simulink model "luenberger_obs2_w_design"  (R2023b)
settings: Solver=FixedStepAuto  StartTime=0.0  StopTime=T  FixedStep=dt  RelTol=1e-3
values from neighbouring files (symbols this model uses):
  A = [0 1 0 -1; -ks/mv -bs/mv 0 bs/mv; 0 0 0 1; ks/mr bs/mr -kp/mr -(bs+bp)/mr]    [define_system.m]
  A_sim_case = eval(sprintf('A_c    [design_cls.m]    (also in design_obs.m)
  B1 = [0; 0; -1; bp/mr]    [define_system.m]
  B1_sim_case = eval(sprintf('B1_c    [design_cls.m]    (also in design_obs.m)
  B2 = [0; 1/mv; 0; -1/mr]    [define_system.m]
  B2_sim_case = eval(sprintf('B2_c    [design_cls.m]    (also in design_obs.m)
  C = [1 0 0 0; -ks/mv -bs/mv 0 bs/mv]    [define_system.m]
  C_obs2 = C(2,:)    [design_cls.m]    (also in design_obs.m)
  C_sim_case = eval(sprintf('C_c    [design_cls.m]    (also in design_obs.m)
  CI = [0; 0; 0; 0]    [design_cls.m]    (also in design_obs.m)
  D = [0; 1/mv]    [define_system.m]
  D_obs2 = D(2)    [design_cls.m]    (also in design_obs.m)
  D_sim_case = eval(sprintf('D_c    [design_cls.m]    (also in design_obs.m)
  Ko = place(A', C_obs2', p_obs2_u)'    [design_cls.m]    (also in design_obs.m; plot_residues.m = place(A', C_', p_obs)')
  T = 32    [design_cls.m]    (also in design_obs.m)
settings Model: Creator=felipe  LastModifiedBy=felipe

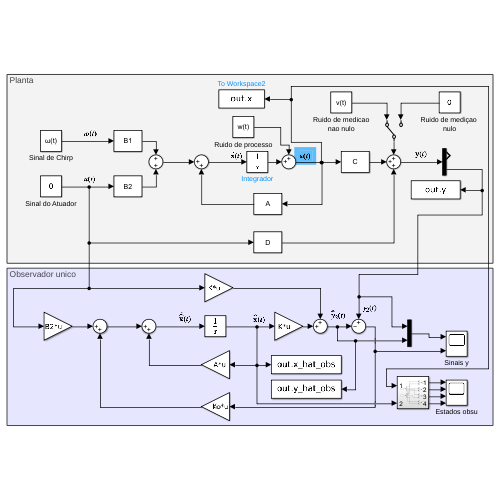
[thumbnail: Simulink's stored preview of the top-level diagram]
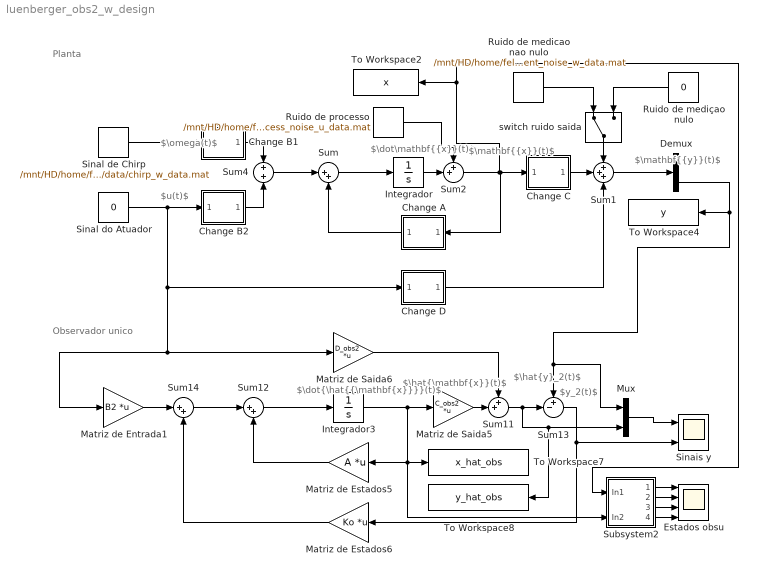
== system luenberger_obs2_w_design ==
  note: Observador unico
  note: $\omega(t)$
  note: Planta
  note: $\dot\mathbf{{x}}(t)$
  note: $\mathbf{{x}}(t)$
  note: $\mathbf{{y}}(t)$
  note: $u(t)$
  note: $\hat{\mathbf{x}}(t)$
  note: $\hat{y}_2(t)$
  note: $y_2(t)$
  note: $\dot{\hat{{\mathbf{x}}}}(t)$
  Change A : Subsystem
      mask Display: disp('A');
  Change B1 : Subsystem
      mask Display: disp('B1');
  Change B2 : Subsystem
      mask Display: disp('B2');
  Change C : Subsystem
      mask Display: disp('C');
  Change D : Subsystem
      mask Display: disp('D');
  Demux : Demux  Outputs=2
  Estados obsu : Scope  NumInputPorts=4
  Integrador : Integrator  InitialCondition=CI
  Integrador3 : Integrator  InitialCondition=CI
  Matriz de Entrada1 : Gain  Gain=B2  Multiplication=Matrix(K*u)
  Matriz de Estados5 : Gain  Gain=A  Multiplication=Matrix(K*u)
  Matriz de Estados6 : Gain  Gain=Ko  Multiplication=Matrix(K*u)
  Matriz de Saida5 : Gain  Gain=C_obs2  Multiplication=Matrix(K*u)
  Matriz de Saida6 : Gain  Gain=D_obs2  Multiplication=Matrix(K*u)
  Mux : Mux  Inputs=2
  Ruido de medicao nao nulo : FromFile  FileName=/mnt/HD/home/felipe/Projects/matlab/TG/data/measurement_noise_w_data.mat  SampleTime=0
      mask Display: disp('v(t)');
  Ruido de mediçao nulo : Constant  Value=0
  Ruido de processo : FromFile  FileName=/mnt/HD/home/felipe/Projects/matlab/TG/data/process_noise_u_data.mat  SampleTime=0
      mask Display: disp('w(t)');
  Sinais y : Scope  NumInputPorts=2
  Sinal de Chirp : FromFile  FileName=/mnt/HD/home/felipe/Projects/matlab/TG/data/chirp_w_data.mat  SampleTime=0
      mask Display: disp('ω(t)');
  Sinal do Atuador : Constant  Value=0
  Subsystem2 : Subsystem
  Sum : Sum  Inputs=|++
  Sum1 : Sum  Inputs=+++
  Sum11 : Sum  Inputs=++|
  Sum12 : Sum  Inputs=|++
  Sum13 : Sum  Inputs=+-|
  Sum14 : Sum  Inputs=|++
  Sum2 : Sum  Inputs=++|
  Sum4 : Sum
  To Workspace2 : ToWorkspace  VariableName=x  SampleTime=-1
  To Workspace4 : ToWorkspace  VariableName=y  SampleTime=-1
  To Workspace7 : ToWorkspace  VariableName=x_hat_obs  SampleTime=-1
  To Workspace8 : ToWorkspace  VariableName=y_hat_obs  SampleTime=-1
  switch ruido saida : ManualSwitch
  wires:
  Change A/1(v_bm) -> Sum/2
  Change B1/1(v_bm) -> Sum4/1
  switch ruido saida/1 -> Sum1/1
  Ruido de mediçao nulo/1 -> switch ruido saida/2
  Ruido de medicao nao nulo/1 -> switch ruido saida/1
  Sum4/1 -> Sum/1
  Change C/1(v_bm) -> Sum1/2
  Integrador/1 -> Sum2/2
  Sum/1 -> Integrador/1
  Change B2/1(v_bm) -> Sum4/2
  Change D/1(v_bm) -> Sum1/3
  Matriz de Entrada1/1 -> Sum14/1
  Matriz de Saida5/1 -> Sum11/2
  Sum14/1 -> Sum12/1
  Subsystem2/1(Out1) -> Estados obsu/1
  Subsystem2/3(Out3) -> Estados obsu/3
  Matriz de Saida6/1 -> Sum11/1
  Integrador3/1 -> Matriz de Saida5/1, To Workspace7/1, Subsystem2/2(In2), Matriz de Estados5/1
  Subsystem2/2(Out2) -> Estados obsu/2
  Sum12/1 -> Integrador3/1
  Subsystem2/4(Out4) -> Estados obsu/4
  Matriz de Estados6/1 -> Sum14/2
  Matriz de Estados5/1 -> Sum12/2
  Sum13/1 -> Sinais y/2, Matriz de Estados6/1
  Sum11/1 -> Mux/2, To Workspace8/1, Sum13/2
  Demux/2 -> To Workspace4/1, Mux/1, Sum13/1
  Sinal do Atuador/1 -> Change B2/1(v_am), Matriz de Saida6/1, Matriz de Entrada1/1, Change D/1(v_am)
  Sinal de Chirp/1 -> Change B1/1(v_am)
  Sum1/1 -> Demux/1
  Mux/1 -> Sinais y/1
  Sum2/1 -> Subsystem2/1(In1), To Workspace2/1, Change C/1(v_am), Change A/1(v_am)
  Ruido de processo/1 -> Sum2/1

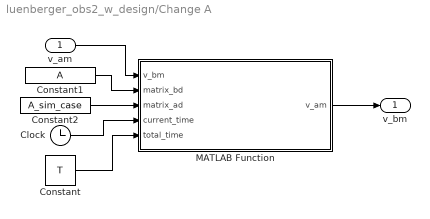
== system luenberger_obs2_w_design/Change A ==
  v_am : Inport
  Clock : Clock
  Constant : Constant  Value=T
  Constant1 : Constant  Value=A
  Constant2 : Constant  Value=A_sim_case
  MATLAB Function : MATLAB Function  TreatAsAtomicUnit=on
  v_bm : Outport
  wires:
  Clock/1 -> MATLAB Function/4(current_time)
  MATLAB Function/1(v_am) -> v_bm/1
  v_am/1 -> MATLAB Function/1(v_bm)
  Constant1/1 -> MATLAB Function/2(matrix_bd)
  Constant/1 -> MATLAB Function/5(total_time)
  Constant2/1 -> MATLAB Function/3(matrix_ad)

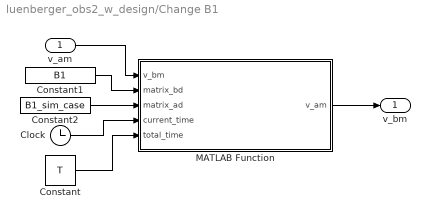
== system luenberger_obs2_w_design/Change B1 ==
  v_am : Inport
  Clock : Clock
  Constant : Constant  Value=T
  Constant1 : Constant  Value=B1
  Constant2 : Constant  Value=B1_sim_case
  MATLAB Function : MATLAB Function  TreatAsAtomicUnit=on
  v_bm : Outport
  wires:
  Clock/1 -> MATLAB Function/4(current_time)
  MATLAB Function/1(v_am) -> v_bm/1
  v_am/1 -> MATLAB Function/1(v_bm)
  Constant1/1 -> MATLAB Function/2(matrix_bd)
  Constant/1 -> MATLAB Function/5(total_time)
  Constant2/1 -> MATLAB Function/3(matrix_ad)

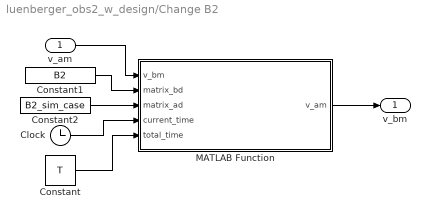
== system luenberger_obs2_w_design/Change B2 ==
  v_am : Inport
  Clock : Clock
  Constant : Constant  Value=T
  Constant1 : Constant  Value=B2
  Constant2 : Constant  Value=B2_sim_case
  MATLAB Function : MATLAB Function  TreatAsAtomicUnit=on
  v_bm : Outport
  wires:
  Clock/1 -> MATLAB Function/4(current_time)
  MATLAB Function/1(v_am) -> v_bm/1
  v_am/1 -> MATLAB Function/1(v_bm)
  Constant1/1 -> MATLAB Function/2(matrix_bd)
  Constant/1 -> MATLAB Function/5(total_time)
  Constant2/1 -> MATLAB Function/3(matrix_ad)

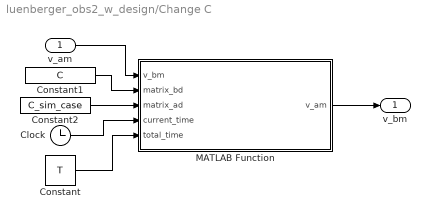
== system luenberger_obs2_w_design/Change C ==
  v_am : Inport
  Clock : Clock
  Constant : Constant  Value=T
  Constant1 : Constant  Value=C
  Constant2 : Constant  Value=C_sim_case
  MATLAB Function : MATLAB Function  TreatAsAtomicUnit=on
  v_bm : Outport
  wires:
  Clock/1 -> MATLAB Function/4(current_time)
  MATLAB Function/1(v_am) -> v_bm/1
  v_am/1 -> MATLAB Function/1(v_bm)
  Constant1/1 -> MATLAB Function/2(matrix_bd)
  Constant/1 -> MATLAB Function/5(total_time)
  Constant2/1 -> MATLAB Function/3(matrix_ad)

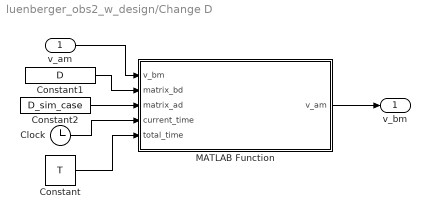
== system luenberger_obs2_w_design/Change D ==
  v_am : Inport
  Clock : Clock
  Constant : Constant  Value=T
  Constant1 : Constant  Value=D
  Constant2 : Constant  Value=D_sim_case
  MATLAB Function : MATLAB Function  TreatAsAtomicUnit=on
  v_bm : Outport
  wires:
  Clock/1 -> MATLAB Function/4(current_time)
  MATLAB Function/1(v_am) -> v_bm/1
  v_am/1 -> MATLAB Function/1(v_bm)
  Constant1/1 -> MATLAB Function/2(matrix_bd)
  Constant/1 -> MATLAB Function/5(total_time)
  Constant2/1 -> MATLAB Function/3(matrix_ad)

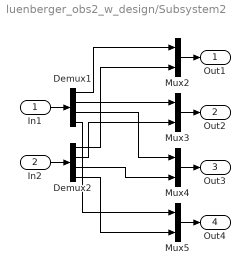
== system luenberger_obs2_w_design/Subsystem2 ==
  In1 : Inport
  In2 : Inport  Port=2
  Demux1 : Demux
  Demux2 : Demux
  Mux{2..5} (4 alike) : Mux  Inputs=2
  Out1 : Outport
  Out2 : Outport  Port=2
  Out3 : Outport  Port=3
  Out4 : Outport  Port=4
  wires:
  Mux5/1 -> Out4/1
  Mux4/1 -> Out3/1
  Mux3/1 -> Out2/1
  Mux2/1 -> Out1/1
  Demux1/3 -> Mux4/1
  Demux2/2 -> Mux3/2
  Demux1/1 -> Mux2/1
  Demux1/2 -> Mux3/1
  In2/1 -> Demux2/1
  Demux2/3 -> Mux4/2
  In1/1 -> Demux1/1
  Demux2/4 -> Mux5/2
  Demux1/4 -> Mux5/1
  Demux2/1 -> Mux2/2

== matlab function luenberger_obs2_w_design/Change B1/MATLAB Function ==
  data: v_bm input; matrix_bd input; matrix_ad input; v_am output; current_time input; total_time input
function v_am = change_matrix(v_bm, matrix_bd, matrix_ad, current_time, total_time)
    if current_time < total_time/2
        v_am = matrix_bd*v_bm;
        return
    end
    v_am = matrix_ad*v_bm;
end

== matlab function luenberger_obs2_w_design/Change D/MATLAB Function ==
  data: v_bm input; matrix_bd input; matrix_ad input; v_am output; current_time input; total_time input
function v_am = change_matrix(v_bm, matrix_bd, matrix_ad, current_time, total_time)
    if current_time < total_time/2
        v_am = matrix_bd*v_bm;
        return
    end
    v_am = matrix_ad*v_bm;
end

== matlab function luenberger_obs2_w_design/Change A/MATLAB Function ==
  data: v_bm input; matrix_bd input; matrix_ad input; v_am output; current_time input; total_time input
function v_am = change_matrix(v_bm, matrix_bd, matrix_ad, current_time, total_time)
    if current_time < total_time/2
        v_am = matrix_bd*v_bm;
        return
    end
    v_am = matrix_ad*v_bm;
end

== matlab function luenberger_obs2_w_design/Change C/MATLAB Function ==
  data: v_bm input; matrix_bd input; matrix_ad input; v_am output; current_time input; total_time input
function v_am = change_matrix(v_bm, matrix_bd, matrix_ad, current_time, total_time)
    if current_time < total_time/2
        v_am = matrix_bd*v_bm;
        return
    end
    v_am = matrix_ad*v_bm;
end

== matlab function luenberger_obs2_w_design/Change B2/MATLAB Function ==
  data: v_bm input; matrix_bd input; matrix_ad input; v_am output; current_time input; total_time input
function v_am = change_matrix(v_bm, matrix_bd, matrix_ad, current_time, total_time)
    if current_time < total_time/2
        v_am = matrix_bd*v_bm;
        return
    end
    v_am = matrix_ad*v_bm;
end
